simulink library "latchHigh_ul"  (R2018b)
settings: Solver=VariableStepAuto  StartTime=0.0  StopTime=10.0  RelTol=1e-3
libraries: simulink x1
settings Model: Creator=mcobb  LastModifiedBy=mcobb

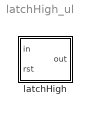
== system latchHigh_ul ==
  latchHigh : Subsystem

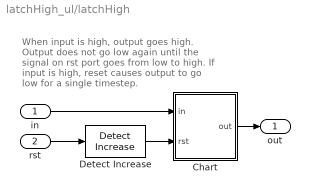
== system latchHigh_ul/latchHigh ==
  note: When input is high, output goes high.
      | Output does not go low again until the
      | signal on rst port goes from low to high.
      | If input is high, reset causes output to
      | go low for a single timestep.
  in : Inport  OutDataTypeStr=boolean  PortDimensions=1
  rst : Inport  Port=2  OutDataTypeStr=boolean  PortDimensions=1
  Chart : Stateflow chart  TreatAsAtomicUnit=on
  Detect Increase : simulink/Logic and Bit Operations/Detect Increase  vinit=false  OutDataTypeStr=boolean
  out : Outport  OutDataTypeStr=boolean  PortDimensions=1
  wires:
  in/1 -> Chart/1(in)
  rst/1 -> Detect Increase/1
  Chart/1(out) -> out/1
  Detect Increase/1 -> Chart/2(rst)

== stateflow chart latchHigh_ul/latchHigh/Chart ==
  state OFF
    out = false;
  state ON
    out = true;
  (default) -> OFF
  ON -> OFF : [rst]
  OFF -> ON : [in]
  data: in input; rst input; out output
